simulink model "Vectors"  (R2025b)
settings: Solver=VariableStepAuto  StartTime=0.0  StopTime=10.0  RelTol=1e-3
settings Model: Creator=Soochan Kim  LastModifiedBy=Soochan Kim

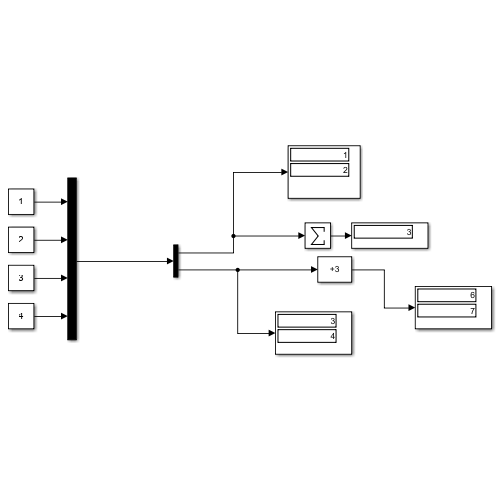
[thumbnail: Simulink's stored preview of the top-level diagram]
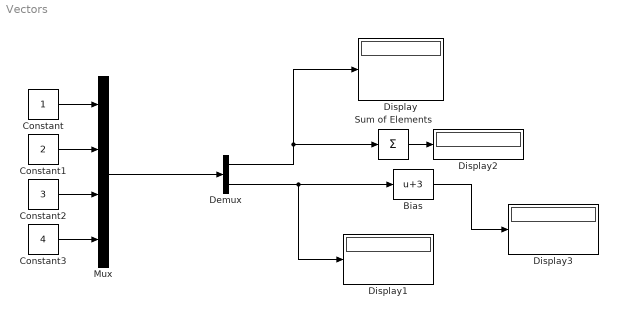
== system Vectors ==
  Bias : Bias  Bias=3  SaturateOnIntegerOverflow=off
  Constant : Constant
  Constant1 : Constant  Value=2
  Constant2 : Constant  Value=3
  Constant3 : Constant  Value=4
  Demux : Demux  Outputs=2
  Display{,1..3} (4 alike) : Display
  Mux : Mux
  Sum of Elements : Sum  Inputs=+
  wires:
  Constant/1 -> Mux/1
  Constant1/1 -> Mux/2
  Constant3/1 -> Mux/4
  Constant2/1 -> Mux/3
  Mux/1 -> Demux/1
  Demux/1 -> Sum of Elements/1, Display/1
  Demux/2 -> Bias/1, Display1/1
  Sum of Elements/1 -> Display2/1
  Bias/1 -> Display3/1
